simulink model "sim_pert_ct"  (R2014b)
settings: Solver=ode45  StartTime=0.0  StopTime=10  RelTol=1e-3
values from neighbouring files (symbols this model uses):
  A = [0 -23.8095;0 0]    [Observador.m]    (also in P1.m; P1_pert.m; P1_pert_range.m; P1_pert_sin.m)
  B = [0;-23.8095]    [Observador.m]    (also in P1.m; P1_pert.m; P1_pert_range.m; P1_pert_sin.m)
  C = [1 0]    [Observador.m]    (also in P1.m; P1_pert.m = eye(2); P1_pert_range.m = eye(2); P1_pert_sin.m = eye(2))
  C_pert = eye(3)    [P1_pert.m]    (also in P1_pert_range.m = eye(5); P1_pert_sin.m = eye(4); P1_pert_sin_ct.m = eye(5); P1_pert_sin_ct_imag.m = eye(5))
  D = [0;0]    [Observador.m]    (also in P1.m; P1_pert.m; P1_pert_range.m; P1_pert_sin.m)
  gam_pert = [gam; 0]    [P1_pert.m]    (also in P1_pert_range.m = [gam; zeros(3,1)]; P1_pert_sin.m = [gam; 0; 0]; P1_pert_sin_ct.m = [gam; 0; 0; 0]; P1_pert_sin_ct_imag.m = [gam; 0; 0; 0])
  K_dis = acker(phi,gam,P_dis)    [Observador.m]    (also in P1.m; P1_pert.m; P1_pert_range.m; P1_pert_sin.m)
  L_pert = K_obs_dis_pert'    [P1_pert.m]    (also in P1_pert_range.m; P1_pert_sin.m; P1_pert_sin_ct.m; P1_pert_sin_ct_imag.m)
  phi_pert = [phi gam; 0 0 1]    [P1_pert.m]    (also in P1_pert_range.m = [phi gam*C_d [0;0]; zeros(2,2) phi_sin [0;0]; zeros(1,4) 1]; P1_pert_sin.m = [phi gam [0;0]; zeros(2) phi_sin]; P1_pert_sin_ct.m = [phi gam gam [0;0]; zeros(3,2) [1;0;0] [[0 0]; phi_sin]]; P1_pert_sin_ct_imag.m = [phi gam gam [0;0]; zeros(3,2) [1;0;0] [[0 0]; phi_sin]])
libraries: simulink x1
settings Model: Creator=student  LastModifiedBy=lluis
settings DataIOCC: SignalLoggingSaveFormat=ModelDataLogs
settings OptimizationCC: ExpressionDepthLimit=2147483647
settings DebuggingCC: UnderspecifiedInitializationDetection=Classic  MergeDetectMultiDrivingBlocksExec=none  FcnCallInpInsideContextMsg=EnableAllAsWarning  StateNameClashWarn=warning
settings GRTTargetCC: CombineOutputUpdateFcns=off  GRTInterface=on

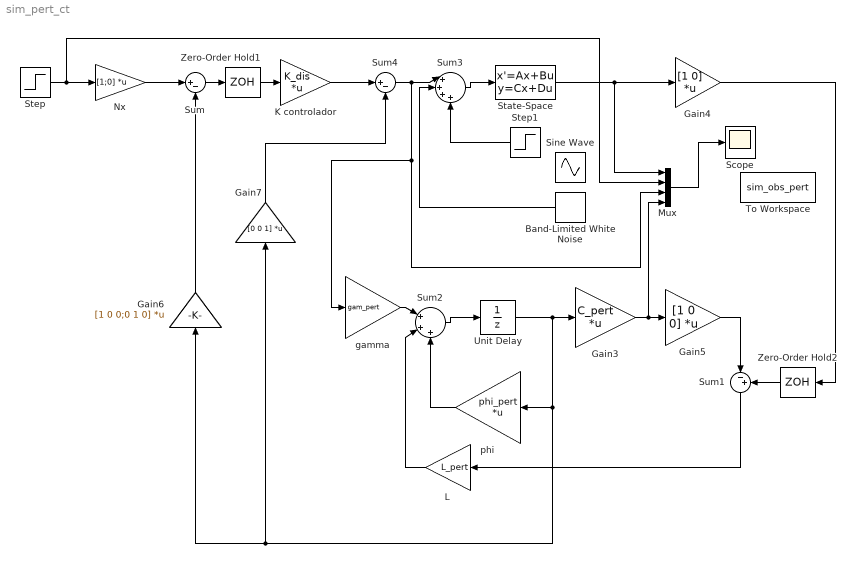
== system sim_pert_ct ==
  Band-Limited White Noise : simulink/Sources/Band-Limited White Noise  Cov=[0.000001]  Ts=0.005  seed=[23341]
  Gain3 : Gain  Gain=C_pert  Multiplication=Matrix(K*u)
  Gain4 : Gain  Gain=[1 0]  Multiplication=Matrix(K*u)
  Gain5 : Gain  Gain=[1 0 0]  Multiplication=Matrix(K*u)
  Gain6 : Gain  Gain=[1 0 0;0 1 0]  Multiplication=Matrix(K*u)
  Gain7 : Gain  Gain=[0 0 1]  Multiplication=Matrix(K*u)
  K controlador : Gain  Gain=K_dis  Multiplication=Matrix(K*u)
  L : Gain  Gain=L_pert
  Mux : Mux
  Nx : Gain  Gain=[1;0]  Multiplication=Matrix(K*u)
  Scope : Scope
  Sine Wave : Sin  Amplitude=0.005  Frequency=15  SampleTime=0
  State-Space : StateSpace  A=A  B=B  C=C  D=D  X0=[1;1]
  Step : Step  SampleTime=0
  Step1 : Step  Time=0  After=-0.05  SampleTime=0
  Sum : Sum  Inputs=|+-
  Sum1 : Sum  Inputs=|-+
  Sum2 : Sum  Inputs=|+++
  Sum3 : Sum  Inputs=|++++
  Sum4 : Sum  Inputs=|+-
  To Workspace : ToWorkspace  VariableName=sim_obs_pert  SaveFormat=Timeseries  SampleTime=-1
  Unit Delay : UnitDelay  SampleTime=-1
  Zero-Order Hold1 : ZeroOrderHold  SampleTime=5E-2
  Zero-Order Hold2 : ZeroOrderHold  SampleTime=5E-2
  gamma : Gain  Gain=gam_pert
  phi : Gain  Gain=phi_pert  Multiplication=Matrix(K*u)
  wires:
  State-Space/1 -> Mux/1, Gain4/1
  Sum/1 -> Zero-Order Hold1/1
  Step/1 -> Mux/2, Nx/1
  Nx/1 -> Sum/1
  Zero-Order Hold1/1 -> K controlador/1
  Gain3/1 -> Mux/4, Gain5/1
  Sum1/1 -> L/1
  gamma/1 -> Sum2/1
  L/1 -> Sum2/2
  Unit Delay/1 -> Gain7/1, Gain6/1, phi/1, Gain3/1
  Sum2/1 -> Unit Delay/1
  phi/1 -> Sum2/3
  Gain4/1 -> Zero-Order Hold2/1
  Gain5/1 -> Sum1/1
  K controlador/1 -> Sum4/1
  Zero-Order Hold2/1 -> Sum1/2
  Sum3/1 -> State-Space/1
  Gain6/1 -> Sum/2
  Sum4/1 -> gamma/1, Mux/3, Sum3/1
  Gain7/1 -> Sum4/2
  Mux/1 -> Scope/1
  Band-Limited White Noise/1 -> Sum3/2
  Step1/1 -> Sum3/4
